simulink model "dc_2"  (Simulink 7.4)
settings: Solver=ode45  StartTime=0.0  StopTime=inf  MaxStep=1/(2*Fc)  RelTol=1e-3
PreLoadFcn:
  | Fc    =  890e6;
  | Fsym=  20e6;
  | Frame=128;
  | D=8;
  | RRC_Delay=8;
undefined symbols (not defined in the file): Fs, sided, Two
libraries: dsparch4 x8, dspbuff3 x4, commdigbbndpm3 x3, commfilt2 x3, simulink x3, commsink2 x2, dspsnks4 x2, commrandsrc2 x2, commrflib2 x1
settings Model: Creator=dbenson  LastModifiedBy=Dick
settings OptimizationCC: InitFltsAndDblsToZero=on

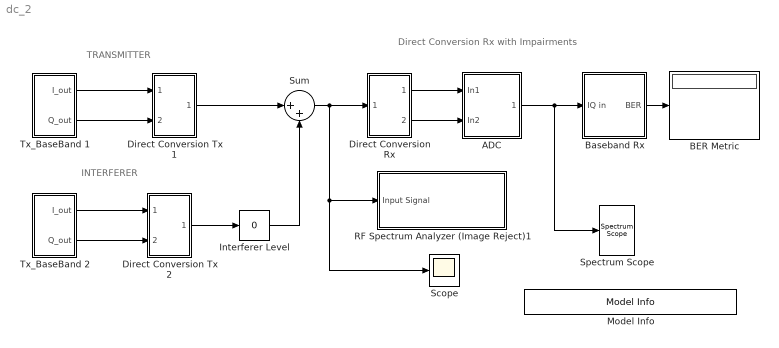
== system dc_2 ==
  note: INTERFERER
  note: TRANSMITTER
  note: Direct Conversion Rx with Impairments
  ADC : Subsystem
  BER Metric : Display
  Baseband Rx : Subsystem
  Direct Conversion Rx : Subsystem
  Direct Conversion Tx 1 : Subsystem
  Direct Conversion Tx 2 : Subsystem
  Interferer Level : simulink/Math Operations/Slider Gain  SystemSampleTime=-1  low=0  gain=0  high=10
  Model Info : simulink/Model-Wide Utilities/Model Info  SystemSampleTime=-1  InitialBlockCM=None  BlockCM=None  Frame=on  DisplayStringWithTags=Copywrite 2005-2010 The MathWorks, Inc.  HorizontalTextAlignment=Center  LeftAlignmentValue=0.5  SourceBlockDiagram=dc_2  TagMaxNumber=20
  RF Spectrum Analyzer (Image Reject)1 : Subsystem  Description=Spectrum Analyzer  mask{BW=100e6, Fc=Fc}
      mask prompts: BW "Bandwidth"; Fc "Center Freq"
      mask Display: fprintf('Spectrum Analyzer \n Fc=%7.2f MHz \n BW=%7.2f MHz',Fc/1e6,BW/1e6)
  Scope : Scope
      settings: TimeRange=5e-007  YMin=-12.5  YMax=12.5
  Spectrum Scope : dspsnks4/Spectrum Scope  DialogController=dspdialog.SpectrumScope  DialogControllerArgs=DataTag3  SystemSampleTime=-1  ScopeProperties=on  Domain=Frequency  HorizSpan=1  UseBuffer=on  BufferSize=256  Overlap=0  inpFftLenInherit=off  FFTlength=128  numAvg=20  DisplayProperties=off  AxisGrid=on  Memory=off  FrameNumber=on  AxisLegend=off  AxisZoom=off  OpenScopeAtSimStart=on  OpenScopeImmediately=off  FigPos=[301 38 356 231]  AxisProperties=off  XUnits=Hertz  XRange=Two-sided ((-Fs/2...Fs/2])  XDisplay=0  InheritXIncr=on  XIncr=1.0  XLabel=Samples  XLimit=Auto  YUnits=dBm  XMax=1  XMin=0  YLabel=dBm  LineProperties=off  wintypeSpecScope=Hann  RsSpecScope=50  betaSpecScope=5  winsampSpecScope=Periodic  XAxisParamsVer=6.8
      settings: YMin=-60  YMax=20
  Sum : Sum  Inputs=|++  OutDataType=sfix(16)  OutScaling=2^0
  Tx_BaseBand 1 : Subsystem
  Tx_BaseBand 2 : Subsystem
  wires:
  Tx_BaseBand 1/1(I_out) -> Direct Conversion Tx 1/1(In1)
  Tx_BaseBand 1/2(Q_out) -> Direct Conversion Tx 1/2(In2)
  ADC/1(I/Q out) -> Baseband Rx/1(IQ in), Spectrum Scope/1
  Direct Conversion Rx/1(Out1) -> ADC/1(In1)
  Direct Conversion Rx/2(Out2) -> ADC/2(In2)
  Baseband Rx/1(BER) -> BER Metric/1
  Direct Conversion Tx 1/1(Out1) -> Sum/1
  Interferer Level/1 -> Sum/2
  Sum/1 -> Direct Conversion Rx/1(In1), RF Spectrum Analyzer (Image Reject)1/1(Input Signal), Scope/1
  Tx_BaseBand 2/1(I_out) -> Direct Conversion Tx 2/1(In1)
  Tx_BaseBand 2/2(Q_out) -> Direct Conversion Tx 2/2(In2)
  Direct Conversion Tx 2/1(Out1) -> Interferer Level/1

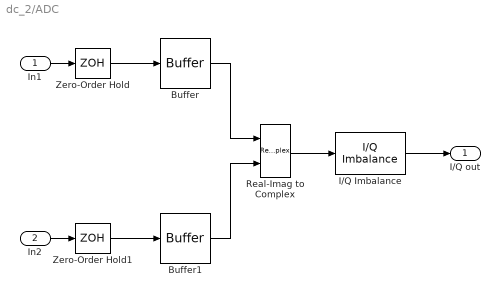
== system dc_2/ADC ==
  In1 : Inport
  In2 : Inport  Port=2
  Buffer : dspbuff3/Buffer  N=Frame*D  V=0  ic=0
  Buffer1 : dspbuff3/Buffer  N=Frame*D  V=0  ic=0
  I/Q Imbalance : commrflib2/I//Q Imbalance  SystemSampleTime=-1  ampImbal=0  phsImbal=0  Idc=0  Qdc=0
  Real-Imag to Complex : RealImagToComplex
  Zero-Order Hold : ZeroOrderHold  SampleTime=1/(D*Fsym)
  Zero-Order Hold1 : ZeroOrderHold  SampleTime=1/(D*Fsym)
  I/Q out : Outport
  wires:
  In1/1 -> Zero-Order Hold/1
  Zero-Order Hold/1 -> Buffer/1
  In2/1 -> Zero-Order Hold1/1
  Zero-Order Hold1/1 -> Buffer1/1
  Buffer/1 -> Real-Imag to Complex/1
  Buffer1/1 -> Real-Imag to Complex/2
  Real-Imag to Complex/1 -> I/Q Imbalance/1
  I/Q Imbalance/1 -> I/Q out/1

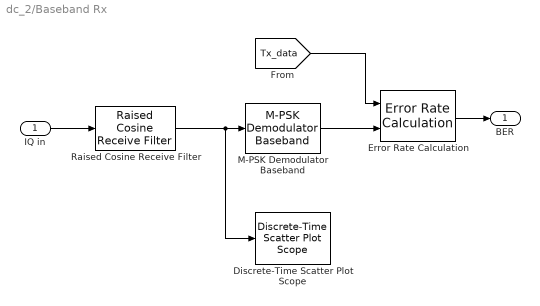
== system dc_2/Baseband Rx ==
  IQ in : Inport
  Discrete-Time Scatter Plot Scope : commsink2/Discrete-Time Scatter Plot Scope  Tag=ScatterPlot  SystemSampleTime=-1  sampPerSymb=1  offsetEye=0  numTraces=40  numNewFrames=40  LineMarkers=.  LineColors=b  fading=off  render=off  AxisGrid=on  xMin=-2.5  xMax=2.5  yMin=-2.5  yMax=2.5  inphaseLabel=In-phase Amplitude  quadratureLabel=Quadrature Amplitude  openScopeAtSimStart=on  FrameNumber=off  FigPos=[750 67 230 238]  figTitle=Scatter Plot  numLinesMax=8  block_type_=scatter
  Error Rate Calculation : commsink2/Error Rate Calculation  N=Frame+2*RRC_Delay  st_delay=0  cp_mode=Entire frame  subframe=[]  PMode=Port  WsName=ErrorVec  RsMode2=off  stop=off  numErr=100  maxBits=1e6
  M-PSK Demodulator Baseband : commdigbbndpm3/M-PSK Demodulator Baseband  DialogController=commDDGCreate  DialogControllerArgs=DataTag0  M=4  Ph=pi/4  Dec=Binary  Mapping=[0:7]  OutType=Integer  DecType=Hard decision  VarSource=Dialog  Variance=1  outDtype1=Inherit via internal rule  outDtype2=Inherit via internal rule  derotateFactorWordLen=16
  Raised Cosine Receive Filter : commfilt2/Raised Cosine Receive Filter  DialogController=dspDDGCreate  DialogControllerArgs=DataTag1  SystemSampleTime=-1  filtType=Square root  N=8  D=RRC_Delay  R=0.25  sampMode=Mute  saveAsFlag=0  framing=Maintain input frame rate  rateMode=Downsampling  downFactor=D  downOffset=6  checkGain=Normalized  filterGain=1  checkCoeff=off  variableName=rcRxFilt  launchFVT=off  roundingMode=Floor  overflowMode=off
  BER : Outport
  wires:
  Raised Cosine Receive Filter/1 -> Discrete-Time Scatter Plot Scope/1, M-PSK Demodulator Baseband/1
  [Tx_data] -> Error Rate Calculation/1
  M-PSK Demodulator Baseband/1 -> Error Rate Calculation/2
  IQ in/1 -> Raised Cosine Receive Filter/1
  Error Rate Calculation/1 -> BER/1

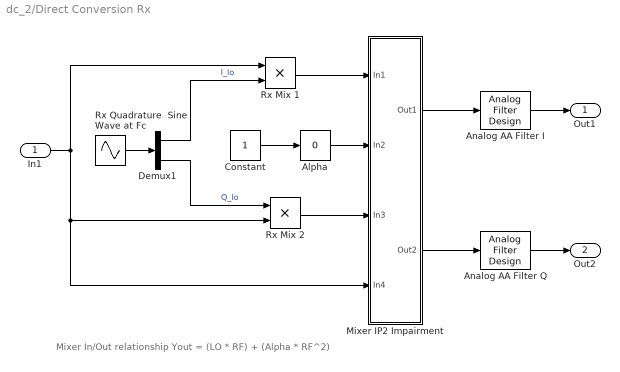
== system dc_2/Direct Conversion Rx ==
  note: Mixer In/Out relationship
      | Yout = (LO * RF) + (Alpha * RF^2)
  In1 : Inport
  Alpha : simulink/Math Operations/Slider Gain  SystemSampleTime=-1  low=0  gain=0  high=0.1
  Analog AA Filter I : dsparch4/Analog Filter Design  method=Bessel  filttype=Lowpass  N=5  Wlo=2*pi*2*Fsym  Whi=80  Rp=2  Rs=40
  Analog AA Filter Q : dsparch4/Analog Filter Design  method=Bessel  filttype=Lowpass  N=5  Wlo=2*pi*2*Fsym  Whi=80  Rp=2  Rs=40
  Constant : Constant  OutDataType=sfix(16)  OutScaling=2^0
  Demux1 : Demux  Outputs=2
  Mixer IP2 Impairment : Subsystem
  Rx Mix 1 : Product  OutDataType=sfix(16)  OutScaling=2^0  RndMeth=Zero
  Rx Mix 2 : Product  OutDataType=sfix(16)  OutScaling=2^0  RndMeth=Zero
  Rx Quadrature  Sine Wave at Fc : Sin  Amplitude=1  Bias=0  Frequency=Fc*2*pi  Phase=[-pi/2,0]  Samples=10  SampleTime=0  Offset=0
  Out1 : Outport
  Out2 : Outport  Port=2
  wires:
  In1/1 -> Rx Mix 1/1, Rx Mix 2/2, Mixer IP2 Impairment/4(In4)
  Rx Quadrature  Sine Wave at Fc/1 -> Demux1/1
  Demux1/1 -> Rx Mix 1/2  "I_lo"
  Demux1/2 -> Rx Mix 2/1  "Q_lo"
  Analog AA Filter I/1 -> Out1/1
  Analog AA Filter Q/1 -> Out2/1
  Rx Mix 1/1 -> Mixer IP2 Impairment/1(In1)
  Alpha/1 -> Mixer IP2 Impairment/2(In2)
  Rx Mix 2/1 -> Mixer IP2 Impairment/3(In3)
  Mixer IP2 Impairment/1(Out1) -> Analog AA Filter I/1
  Mixer IP2 Impairment/2(Out2) -> Analog AA Filter Q/1
  Constant/1 -> Alpha/1

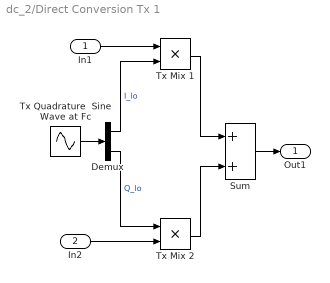
== system dc_2/Direct Conversion Tx 1 ==
  In1 : Inport
  In2 : Inport  Port=2
  Demux : Demux  Outputs=2
  Sum : Sum  OutDataType=sfix(16)  OutScaling=2^0
  Tx Mix 1 : Product  OutDataType=sfix(16)  OutScaling=2^0  RndMeth=Zero
  Tx Mix 2 : Product  OutDataType=sfix(16)  OutScaling=2^0  RndMeth=Zero
  Tx Quadrature  Sine Wave at Fc : Sin  Amplitude=4.1  Bias=0  Frequency=Fc*2*pi  Phase=[-pi/2,0]  Samples=10  SampleTime=0  Offset=0
  Out1 : Outport
  wires:
  Tx Quadrature  Sine Wave at Fc/1 -> Demux/1
  Demux/1 -> Tx Mix 1/2  "I_lo"
  Demux/2 -> Tx Mix 2/1  "Q_lo"
  Tx Mix 1/1 -> Sum/1
  Tx Mix 2/1 -> Sum/2
  In1/1 -> Tx Mix 1/1
  Sum/1 -> Out1/1
  In2/1 -> Tx Mix 2/2

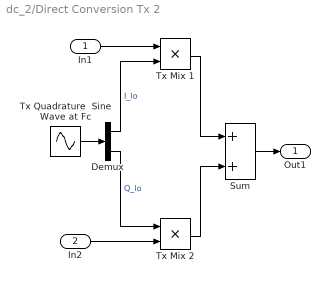
== system dc_2/Direct Conversion Tx 2 ==
  In1 : Inport
  In2 : Inport  Port=2
  Demux : Demux  Outputs=2
  Sum : Sum  OutDataType=sfix(16)  OutScaling=2^0
  Tx Mix 1 : Product  OutDataType=sfix(16)  OutScaling=2^0  RndMeth=Zero
  Tx Mix 2 : Product  OutDataType=sfix(16)  OutScaling=2^0  RndMeth=Zero
  Tx Quadrature  Sine Wave at Fc : Sin  Amplitude=4.1  Bias=0  Frequency=(Fc+30.0e6)*2*pi  Phase=[-pi/2,0]  Samples=10  SampleTime=0  Offset=0
  Out1 : Outport
  wires:
  In2/1 -> Tx Mix 2/2
  Sum/1 -> Out1/1
  In1/1 -> Tx Mix 1/1
  Tx Mix 2/1 -> Sum/2
  Tx Mix 1/1 -> Sum/1
  Demux/2 -> Tx Mix 2/1  "Q_lo"
  Demux/1 -> Tx Mix 1/2  "I_lo"
  Tx Quadrature  Sine Wave at Fc/1 -> Demux/1

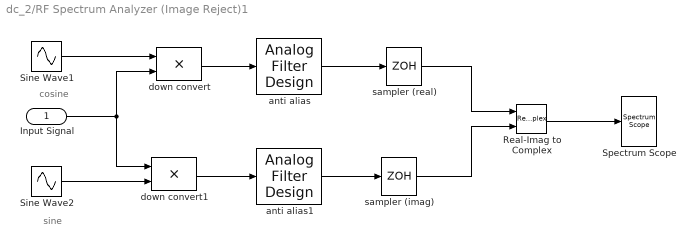
== system dc_2/RF Spectrum Analyzer (Image Reject)1 ==
  note: cosine
  note: sine
  Input Signal : Inport  OutDataType=sfix(16)  OutScaling=2^0
  Real-Imag to Complex : RealImagToComplex
  Sine Wave1 : Sin  Amplitude=1/7.2  Bias=0  Frequency=2*pi*(Fc)  Phase=-pi/2  Samples=10  SampleTime=0  Offset=0
  Sine Wave2 : Sin  Amplitude=1/7.2  Bias=0  Frequency=2*pi*(Fc)  Phase=0  Samples=10  SampleTime=0  Offset=0
  Spectrum Scope : dspsnks4/Spectrum Scope  DialogController=dspdialog.SpectrumScope  DialogControllerArgs=DataTag2  SystemSampleTime=-1  ScopeProperties=on  Domain=Frequency  HorizSpan=1  UseBuffer=on  BufferSize=256  Overlap=0  inpFftLenInherit=off  FFTlength=128  numAvg=20  DisplayProperties=off  AxisGrid=on  Memory=off  FrameNumber=on  AxisLegend=off  AxisZoom=off  OpenScopeAtSimStart=on  OpenScopeImmediately=off  FigPos=[10 31 298 242]  AxisProperties=off  XUnits=Hertz  XRange=Two-sided ((-Fs/2...Fs/2])  XDisplay=0  InheritXIncr=on  XIncr=1.0  XLabel=Samples  XLimit=Auto  YUnits=dBm  XMax=1  XMin=0  YLabel=dBm  LineProperties=off  wintypeSpecScope=Hann  RsSpecScope=50  betaSpecScope=5  winsampSpecScope=Periodic  XAxisParamsVer=6.8
      settings: YMin=-60  YMax=0
  anti alias : dsparch4/Analog Filter Design  method=Elliptic  filttype=Lowpass  N=9  Wlo=BW*pi  Whi=80  Rp=1.2  Rs=100
  anti alias1 : dsparch4/Analog Filter Design  method=Elliptic  filttype=Lowpass  N=9  Wlo=BW*pi  Whi=80  Rp=1.2  Rs=100
  down convert : Product  OutDataType=sfix(16)  OutScaling=2^0  SaturateOnIntegerOverflow=on  InputSameDT=on  OutDataTypeStr=Inherit: Same as first input
  down convert1 : Product  OutDataType=sfix(16)  OutScaling=2^0  SaturateOnIntegerOverflow=on  InputSameDT=on  OutDataTypeStr=Inherit: Same as first input
  sampler (imag) : ZeroOrderHold  SampleTime=1/(1.28*BW)
  sampler (real) : ZeroOrderHold  SampleTime=1/(1.28*BW)
  wires:
  Input Signal/1 -> down convert/2, down convert1/1
  down convert/1 -> anti alias/1
  anti alias/1 -> sampler (real)/1
  Sine Wave1/1 -> down convert/1
  Sine Wave2/1 -> down convert1/2
  anti alias1/1 -> sampler (imag)/1
  down convert1/1 -> anti alias1/1
  sampler (real)/1 -> Real-Imag to Complex/1
  sampler (imag)/1 -> Real-Imag to Complex/2
  Real-Imag to Complex/1 -> Spectrum Scope/1

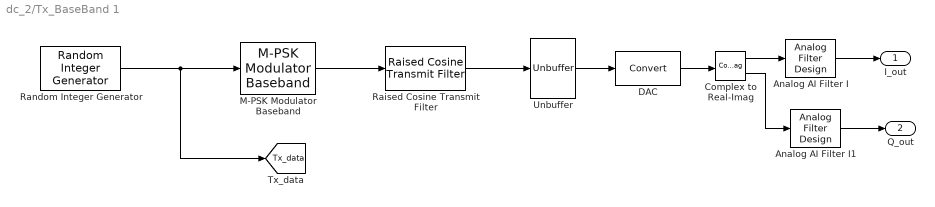
== system dc_2/Tx_BaseBand 1 ==
  Analog AI Filter I : dsparch4/Analog Filter Design  method=Bessel  filttype=Lowpass  N=6  Wlo=2*pi*2*Fsym  Whi=80  Rp=2  Rs=40
  Analog AI Filter I1 : dsparch4/Analog Filter Design  method=Bessel  filttype=Lowpass  N=6  Wlo=2*pi*2*Fsym  Whi=80  Rp=2  Rs=40
  Complex to Real-Imag : ComplexToRealImag
  DAC : DataTypeConversion  OutDataType=sfix(16)  OutScaling=2^0  SampleTime=0
  M-PSK Modulator Baseband : commdigbbndpm3/M-PSK Modulator Baseband  DialogController=commDDGCreate  DialogControllerArgs=DataTag4  M=4  InType=Integer  Enc=Binary  Mapping=[0:7]  Ph=pi/4  outDtype=double  outWordLen=16  outUDDataType=sfix(16)  outFracLenMode=Best precision  outFracLen=15
  Raised Cosine Transmit Filter : commfilt2/Raised Cosine Transmit Filter  DialogController=dspDDGCreate  DialogControllerArgs=DataTag5  SystemSampleTime=-1  filtType=Square root  D=RRC_Delay  R=0.25  sampMode=Mute  saveAsFlag=0  framing=Maintain input frame rate  N=D  checkGain=Normalized  filterGain=1  checkCoeff=off  variableName=rcTxFilt  launchFVT=off  roundingMode=Floor  overflowMode=off
  Random Integer Generator : commrandsrc2/Random Integer Generator  SystemSampleTime=-1  mul=4  seed=37  Ts=1/Fsym  frameBased=on  sampPerFrame=Frame  orient=off  outDataType=double
  Unbuffer : dspbuff3/Unbuffer  ic=0
  I_out : Outport
  Q_out : Outport  Port=2
  tag scope: Tx_data=global
  wires:
  M-PSK Modulator Baseband/1 -> Raised Cosine Transmit Filter/1
  Raised Cosine Transmit Filter/1 -> Unbuffer/1
  Complex to Real-Imag/1 -> Analog AI Filter I/1
  Complex to Real-Imag/2 -> Analog AI Filter I1/1
  Unbuffer/1 -> DAC/1
  DAC/1 -> Complex to Real-Imag/1
  Random Integer Generator/1 -> M-PSK Modulator Baseband/1, [Tx_data]
  Analog AI Filter I/1 -> I_out/1
  Analog AI Filter I1/1 -> Q_out/1

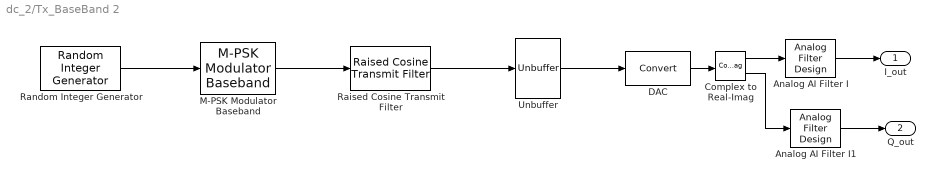
== system dc_2/Tx_BaseBand 2 ==
  Analog AI Filter I : dsparch4/Analog Filter Design  method=Bessel  filttype=Lowpass  N=6  Wlo=2*pi*2*Fsym  Whi=80  Rp=2  Rs=40
  Analog AI Filter I1 : dsparch4/Analog Filter Design  method=Bessel  filttype=Lowpass  N=6  Wlo=2*pi*2*Fsym  Whi=80  Rp=2  Rs=40
  Complex to Real-Imag : ComplexToRealImag
  DAC : DataTypeConversion  OutDataType=sfix(16)  OutScaling=2^0  SampleTime=0
  M-PSK Modulator Baseband : commdigbbndpm3/M-PSK Modulator Baseband  DialogController=commDDGCreate  DialogControllerArgs=DataTag6  M=4  InType=Integer  Enc=Binary  Mapping=[0:7]  Ph=pi/4  outDtype=double  outWordLen=16  outUDDataType=sfix(16)  outFracLenMode=Best precision  outFracLen=15
  Raised Cosine Transmit Filter : commfilt2/Raised Cosine Transmit Filter  DialogController=dspDDGCreate  DialogControllerArgs=DataTag7  SystemSampleTime=-1  filtType=Square root  D=RRC_Delay  R=0.25  sampMode=Mute  saveAsFlag=0  framing=Maintain input frame rate  N=D  checkGain=Normalized  filterGain=1  checkCoeff=off  variableName=rcTxFilt  launchFVT=off  roundingMode=Floor  overflowMode=off
  Random Integer Generator : commrandsrc2/Random Integer Generator  SystemSampleTime=-1  mul=4  seed=123  Ts=1/Fsym  frameBased=on  sampPerFrame=Frame  orient=off  outDataType=double
  Unbuffer : dspbuff3/Unbuffer  ic=0
  I_out : Outport
  Q_out : Outport  Port=2
  wires:
  Analog AI Filter I1/1 -> Q_out/1
  Analog AI Filter I/1 -> I_out/1
  Random Integer Generator/1 -> M-PSK Modulator Baseband/1
  DAC/1 -> Complex to Real-Imag/1
  Unbuffer/1 -> DAC/1
  Complex to Real-Imag/2 -> Analog AI Filter I1/1
  Complex to Real-Imag/1 -> Analog AI Filter I/1
  Raised Cosine Transmit Filter/1 -> Unbuffer/1
  M-PSK Modulator Baseband/1 -> Raised Cosine Transmit Filter/1

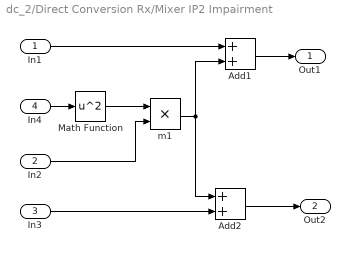
== system dc_2/Direct Conversion Rx/Mixer IP2 Impairment ==
  In1 : Inport
  In2 : Inport  Port=2
  In3 : Inport  Port=3
  In4 : Inport  Port=4
  Add1 : Sum  OutDataType=sfix(16)  OutScaling=2^-10
  Add2 : Sum  OutDataType=sfix(16)  OutScaling=2^-10
  Math Function : Math  Operator=square  OutDataType=sfix(16)  OutScaling=2^0  SaturateOnIntegerOverflow=on
  m1 : Product  OutDataType=sfix(16)  OutScaling=2^0  RndMeth=Zero
  Out1 : Outport
  Out2 : Outport  Port=2
  wires:
  Math Function/1 -> m1/1
  In1/1 -> Add1/1
  m1/1 -> Add1/2, Add2/1
  In3/1 -> Add2/2
  In2/1 -> m1/2
  Add1/1 -> Out1/1
  Add2/1 -> Out2/1
  In4/1 -> Math Function/1
